simulink model "PAM2_example"  (Simulink 7.8)
settings: Solver=VariableStepDiscrete  StartTime=0.0  StopTime=2*Tdur  RelTol=1e-6
PreLoadFcn:
  | clc;
  | clear all;
  | close all;
  | %-------------------
  | Eh = 1;
  | EsNo = 10;
  | %-------------------
  | Rs =  1000;   % bps
  | adc = 8;
  | %-------------------
  | rr = 0.35;
  | GD = 5;        % Group delay
  | Nup = 4;       % Upsampling
  | 
  | Nsymbols = 1024;
  | Nsamples=Nsymbols*Nup;
  | Tdur = Nsymbols/Rs;
StartFcn:
  | %s = serial('COM1','BaudRate',19200,'Parity','even', 'Terminator', '');
  | %fopen(s)
StopFcn:
  | %fclose(s)
  | %delete(s)
  | %clear s
libraries: commdigbbndam3 x2, commfilt2 x2, simulink_need_slupdate x2, commchan3 x1, commrandsrc2 x1, commsink2 x1
settings Model: Creator=theodore  LastModifiedBy=theodore
settings OptimizationCC: InlineInvariantSignals=on  InitFltsAndDblsToZero=on
settings DebuggingCC: SaveWithParameterizedLinksMsg=none  SignalResolutionControl=TryResolveAllWithWarning  MultiTaskDSMMsg=warning  MultiTaskCondExecSysMsg=none  FcnCallInpInsideContextMsg=Use local settings  StrictBusMsg=None
settings RTWCC: IncludeERTFirstTime=on
settings GRTTargetCC: TargetFcnLib=ansi_tfl_tmw.mat

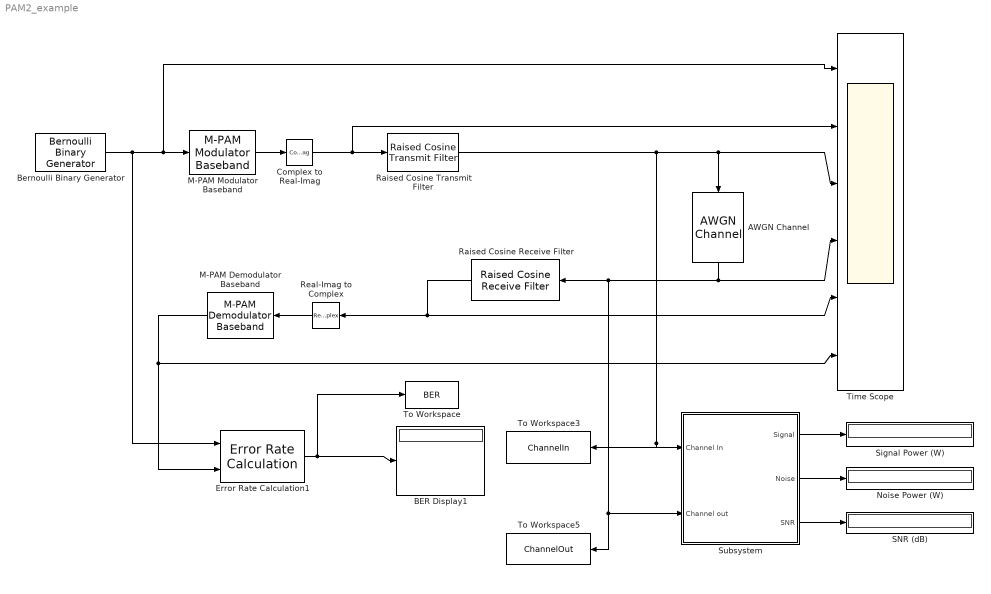
== system PAM2_example ==
  AWGN Channel : commchan3/AWGN Channel  InputProcessing=Columns as channels (frame based)  seed=67  noiseMode="Signal to noise ratio  (Es/No)"  EbNodB=10  EsNodB=EsNo  SNRdB=10  bitsPerSym=1  Ps=1  Tsym=1/(Nup*Rs)  variance=1
  BER Display1 : Display
  Bernoulli Binary Generator : commrandsrc2/Bernoulli Binary Generator  P=0.5  seed=61  Ts=1/Rs  frameBased=off  sampPerFrame=1  orient=off  outDataType=double
  Complex to Real-Imag : ComplexToRealImag  Output=Real
  Error Rate Calculation1 : commsink2/Error Rate Calculation  N=2*GD  st_delay=20  cp_mode=Entire frame  subframe=[]  PMode=Port  WsName=BER  RsMode2=off  stop=off  numErr=100  maxBits=1000
  M-PAM Demodulator Baseband : commdigbbndam3/M-PAM Demodulator Baseband  M=2  OutType=Bit  Dec=Gray  PowType=Min. distance between symbols  MinDist=2  AvgPow=1  PeakPow=1  outDtype1=Inherit via internal rule  outDtype2=Inherit via internal rule  denormFactorWordLen=16  prodOutWordLen=16  prodOutRoundingMode=Floor  prodOutOverflowMode=Wrap  sumWordLen=16
  M-PAM Modulator Baseband : commdigbbndam3/M-PAM Modulator Baseband  M=2  InType=Bit  Enc=Gray  PowType=Min. distance between symbols  MinDist=2  AvgPow=1  PeakPow=1  outDtype=double  outWordLen=16  outUDDataType=sfix(16)  outFracLenMode=Best precision  outFracLen=15
  Noise Power (W) : Display
      settings: Decimation=32
  Raised Cosine Receive Filter : commfilt2/Raised Cosine Receive Filter  filtType=Square root  N=Nup  D=GD  R=rr  sampMode=Mute  saveAsFlag=0  rateMode=Downsampling  downFactor=Nup  downOffset=0  framing=Allow multirate processing  checkGain=User-specified  filterGain=0.5  checkCoeff=on  variableName=rcRxFilt  launchFVT=off  roundingMode=Floor  overflowMode=off
  Raised Cosine Transmit Filter : commfilt2/Raised Cosine Transmit Filter  filtType=Square root  D=GD  R=rr  sampMode=Mute  saveAsFlag=0  N=Nup  framing=Allow multirate processing  checkGain=User-specified  filterGain=2  checkCoeff=on  variableName=rcTxFilt  launchFVT=off  roundingMode=Floor  overflowMode=off
  Real-Imag to Complex : RealImagToComplex  Input=Real
  SNR (dB) : Display
      settings: Decimation=32
  "Signal Power (W)  " : Display
      settings: Decimation=32
  Subsystem : Subsystem
  Time Scope : Scope  NumInputPorts=6
      settings: TimeRange=2.5  YMin=-0.1~-4~-2~-2~-2~-0.5  YMax=1.1~4~2~2~2~1.5  DataFormat=Structure
  To Workspace : ToWorkspace  VariableName=BER  SampleTime=-1  SaveFormat=Array
  To Workspace3 : ToWorkspace  VariableName=ChannelIn  SampleTime=-1  SaveFormat=Array
  To Workspace5 : ToWorkspace  VariableName=ChannelOut  SampleTime=-1  SaveFormat=Array
  wires:
  Bernoulli Binary Generator/1 -> M-PAM Modulator Baseband/1, Time Scope/1, Error Rate Calculation1/1
  Complex to Real-Imag/1 -> Raised Cosine Transmit Filter/1, Time Scope/2
  M-PAM Demodulator Baseband/1 -> Time Scope/6, Error Rate Calculation1/2
  Error Rate Calculation1/1 -> BER Display1/1, To Workspace/1
  Raised Cosine Transmit Filter/1 -> AWGN Channel/1, Time Scope/3, Subsystem/1(Channel In), To Workspace3/1
  Raised Cosine Receive Filter/1 -> Real-Imag to Complex/1, Time Scope/5
  AWGN Channel/1 -> Time Scope/4, Raised Cosine Receive Filter/1, Subsystem/2(Channel out), To Workspace5/1
  M-PAM Modulator Baseband/1 -> Complex to Real-Imag/1
  Real-Imag to Complex/1 -> M-PAM Demodulator Baseband/1
  Subsystem/1(Signal) -> "Signal Power (W)  "/1
  Subsystem/2(Noise) -> Noise Power (W)/1
  Subsystem/3(SNR) -> SNR (dB)/1

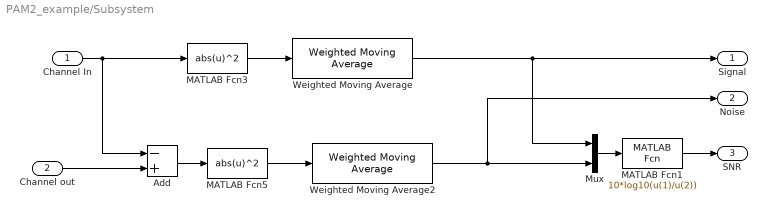
== system PAM2_example/Subsystem ==
  Channel In : Inport
  Channel out : Inport  Port=2
  Add : Sum  Inputs=-+
  MATLAB Fcn1 : MATLABFcn  MATLABFcn=10*log10(u(1)/u(2))
  MATLAB Fcn3 : MATLABFcn  MATLABFcn=abs(u)^2
  MATLAB Fcn5 : MATLABFcn  MATLABFcn=abs(u)^2
  Mux : Mux  Inputs=2
  Weighted Moving Average : simulink_need_slupdate/Weighted Moving Average  mgainval=ones(1, Nsamples)/Nsamples  vinit=0.0  samptime=-1  OutDataType=sfix(16)  OutScaling=2^-10  DoSatur=off  GainDataType=sfix( 16 )  MatRadixGroup=Best Precision: Matrix-wise  GainScaling=2^-10
  Weighted Moving Average2 : simulink_need_slupdate/Weighted Moving Average  mgainval=ones(1, Nsamples)/Nsamples  vinit=0.0  samptime=-1  OutDataType=sfix(16)  OutScaling=2^-10  DoSatur=off  GainDataType=sfix( 16 )  MatRadixGroup=Best Precision: Matrix-wise  GainScaling=2^-10
  Signal : Outport
  Noise : Outport  Port=2
  SNR : Outport  Port=3
  wires:
  Channel In/1 -> Add/1, MATLAB Fcn3/1
  Channel out/1 -> Add/2
  MATLAB Fcn3/1 -> Weighted Moving Average/1
  MATLAB Fcn5/1 -> Weighted Moving Average2/1
  Add/1 -> MATLAB Fcn5/1
  Weighted Moving Average/1 -> Signal/1, Mux/1
  Weighted Moving Average2/1 -> Noise/1, Mux/2
  MATLAB Fcn1/1 -> SNR/1
  Mux/1 -> MATLAB Fcn1/1
